simulink model "filrSimulink"  (R2014a)
settings: Solver=ode45  StartTime=0.0  StopTime=10.0  RelTol=1e-3
values from neighbouring files (symbols this model uses):
  A = 9    [esercizio.m]
libraries: cstblocks x2, simulink x2
settings Model: Creator=User  LastModifiedBy=User

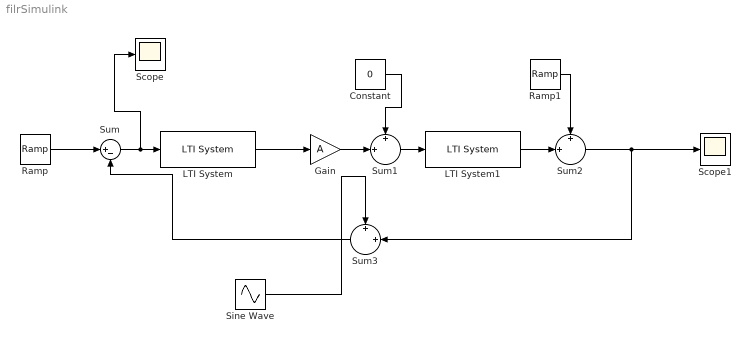
== system filrSimulink ==
  Constant : Constant  Value=0
  Gain : Gain  Gain=A
  LTI System : cstblocks/LTI System  sys=C  IC=[]
  LTI System1 : cstblocks/LTI System  sys=F  IC=[]
  Ramp : simulink/Sources/Ramp  slope=0  start=0  X0=0
  Ramp1 : simulink/Sources/Ramp  slope=0  start=0  X0=0
  Scope : Scope
  Scope1 : Scope
  Sine Wave : Sin  Amplitude=10^-3  Frequency=30  SampleTime=0
  Sum : Sum  Inputs=|+-
  Sum1 : Sum  Inputs=+|+||
  Sum2 : Sum  Inputs=+|+||
  Sum3 : Sum  Inputs=+|+||
  wires:
  Ramp/1 -> Sum/1
  Sum/1 -> Scope/1, LTI System/1
  LTI System/1 -> Gain/1
  Gain/1 -> Sum1/2
  Sum1/1 -> LTI System1/1
  LTI System1/1 -> Sum2/2
  Ramp1/1 -> Sum2/1
  Sum2/1 -> Sum3/2, Scope1/1
  Constant/1 -> Sum1/1
  Sum3/1 -> Sum/2
  Sine Wave/1 -> Sum3/1
